simulink model "test"  (R2021a)
settings: Solver=FixedStepAuto  StartTime=0.0  StopTime=10  RelTol=1e-3
InitFcn:
  | load('BusDefinitions.mat')
values from neighbouring files (symbols this model uses):
  M = [2.03476350051e-06 9.69056117119e-08 9.69056117119e-08 -1.05662818468e-08 2.03476350051e-06 -9.69056117119e-08 9.69056117119e-08 1.05662818468e-08 2.03476350051e-06 -9.69056117119e-08 -9.69056117119e-08 -1.05662818468e-08 ... (16 elements, 4x4)]    [RSdata_Kalman.mat]
undefined symbols (not defined in the file or in its folder): codertarget, Ts, W
settings Model: ExtModeTrigDuration=80  Creator=tomwh  LastModifiedBy=tomwh
settings SolverCC: AlgebraicLoopSolver=TrustRegion
settings OptimizationCC: PassReuseOutputArgsThreshold=0  MaxStackSize=64
settings DebuggingCC: ParameterTunabilityLossMsg=error  SFMachineParentedDataDiag=warning  ArithmeticOperatorsInVariantConditions=warning
settings HardwareCC: ProdBitPerPointer=32  ProdBitPerSizeT=32  ProdBitPerPtrDiffT=32  ProdLargestAtomicInteger=Long  ProdWordSize=32  ProdHWDeviceType=ARM Compatible->ARM 9  UseEmbeddedCoderFeatures=off
settings SFSimCC: SimUseLocalCustomCode=off  MATLABDynamicMemAlloc=off
settings RTWCC: SystemTargetFile=ert.tlc  HardwareBoard=PARROT Mambo  TLCOptions="-aInlineSetEventsForThisBaseRateFcn=TLC_FALSE -aSuppressMultiTaskScheduler=TLC_FALSE   -aRateBasedStepFcn=1"  TemplateMakefile=ert_default_tmf  GenerateReport=on  RTWUseLocalCustomCode=off  Toolchain=Sourcery G++ Lite GNU Toolchain for Drones  LaunchReport=on
settings CodeAppCC: ForceParamTrailComments=on  OperatorAnnotations=on  StateflowObjectComments=on
settings ERTTargetCC: ERTCustomFileBanners=off  MatFileLogging=on  SupportContinuousTime=on  SupportNonInlinedSFcns=on  RemoveResetFunc=off  ModelStepFunctionPrototypeControlCompliant=off

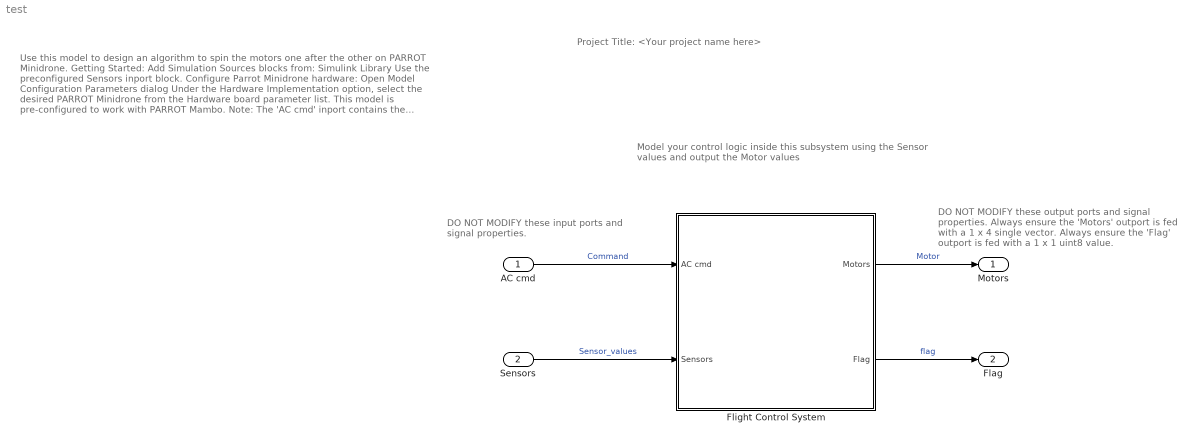
== system test ==
  note: Model your control logic inside this subsystem
      | using the Sensor values and output the
      | Motor values
  note: DO NOT MODIFY these output ports
      | and signal properties.
      |
      |
      |
      | Always ensure the 'Motors' outport
      | is fed with a 1 x 4 single vector.
      |
      |
      |
      |
      |
      | Always ensure the 'Flag' outport is
      | fed with a 1 x 1 uint8 value.
  note: DO NOT MODIFY these input
      | ports and signal properties.
  note: Use this model to design an algorithm to spin the motors one
      | after the other on PARROT Minidrone.
      |
      | Getting Started:
      |
      | Add Simulation Sources blocks from:
      | Simulink Library
      | Use the preconfigured Sensors inport block.
      |
      | Configure Parrot Minidrone hardware:
      |
      | Open Model Configuration Parameters dialog
      |
      | Under the Hardware Implementation option, select the desired
      | PARROT Minidrone from the Hardware board parameter list.
      |
      | This model is pre-configured to work with PARROT Mambo.
      |
      | Note:
      |
      | The 'AC cmd' inport contains the position and orientation
      | reference signals information.
      | The 'Sensors' inport contains data from accelerometer,
      | gyroscope, ultrasonic, pressure and optical flow data.
      | The 'Flag' outport can be used to model an error condition
      | which stops the drone.
      | The 'Motors' outport is fed with the speed values of the 4 motors.
      | Learn more:
      |
      | Simulink Subsystem
      | Simulink Buses
  note: Project Title: <Your project name here>
  AC cmd : Inport  OutDataTypeStr=Bus: CommandBus  BusOutputAsStruct=on
  Sensors : Inport  Port=2  OutDataTypeStr=Bus: SensorsBus  BusOutputAsStruct=on
  Flight Control System : Subsystem  InitFcn=codertarget.parrot.internal.fcsSubsystemCallback(gcb);
  Motors : Outport  OutDataTypeStr=single  PortDimensions=[1 4]  VectorParamsAs1DForOutWhenUnconnected=off
  Flag : Outport  Port=2  OutDataTypeStr=uint8  PortDimensions=1  VectorParamsAs1DForOutWhenUnconnected=off
  wires:
  Flight Control System/1(Motors) -> Motors/1  "Motor"
  AC cmd/1 -> Flight Control System/1(AC cmd)  "Command"
  Sensors/1 -> Flight Control System/2(Sensors)  "Sensor_values"
  Flight Control System/2(Flag) -> Flag/1  "flag"

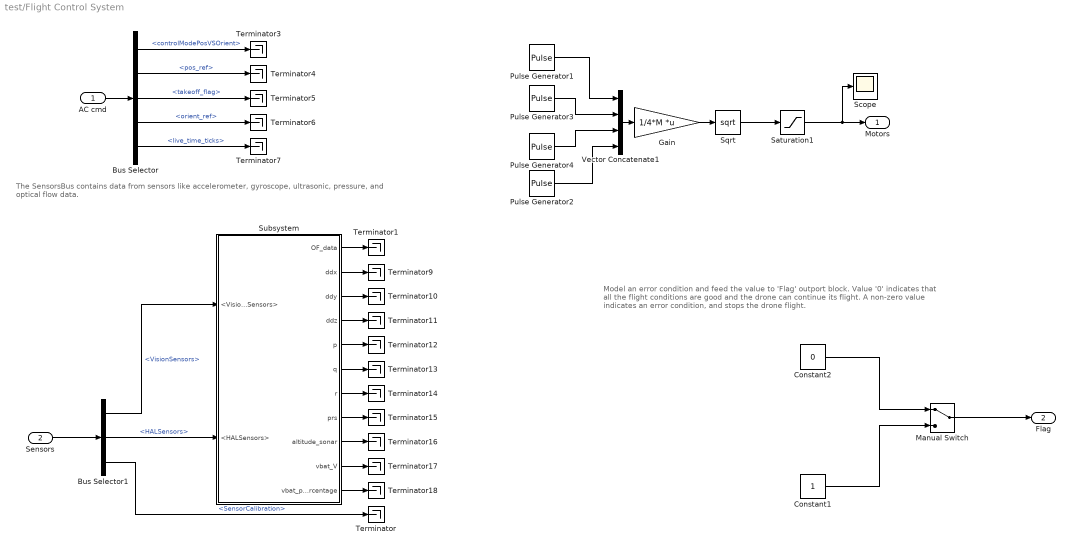
== system test/Flight Control System ==
  note: Model an error condition and feed the value to 'Flag' outport block.
      | Value '0' indicates that all the flight conditions are good and the drone
      | can continue its flight.
      | A non-zero value indicates an error condition, and stops the drone
      | flight.
  note: The SensorsBus contains data from sensors like
      | accelerometer, gyroscope, ultrasonic, pressure,
      | and optical flow data.
  AC cmd : Inport
  Sensors : Inport  Port=2
  Bus Selector : BusSelector  OutputSignals=controlModePosVSOrient,pos_ref,takeoff_flag,orient_ref,live_time_ticks
  Bus Selector1 : BusSelector  OutputSignals=VisionSensors,HALSensors,SensorCalibration
  Constant1 : Constant  OutDataTypeStr=uint8
  Constant2 : Constant  Value=0  OutDataTypeStr=uint8
  Gain : Gain  Gain=1/4*M  Multiplication=Matrix(K*u)
  Manual Switch : ManualSwitch
  Pulse Generator1 : DiscretePulseGenerator  Amplitude=W(1)  Period=1600  PulseWidth=400  SampleTime=Ts
  Pulse Generator2 : DiscretePulseGenerator  Amplitude=W(4)  Period=1600  PulseWidth=400  PhaseDelay=1200  SampleTime=Ts
  Pulse Generator3 : DiscretePulseGenerator  Amplitude=W(2)  Period=1600  PulseWidth=400  PhaseDelay=400  SampleTime=Ts
  Pulse Generator4 : DiscretePulseGenerator  Amplitude=W(3)  Period=1600  PulseWidth=400  PhaseDelay=800  SampleTime=Ts
  Saturation1 : Saturate  UpperLimit=500  LowerLimit=0  OutDataTypeStr=single
  Scope : Scope
  Sqrt : Sqrt  SaturateOnIntegerOverflow=on
  Subsystem : Subsystem
  Terminator{,1,3..7,9..18} (17 alike) : Terminator
  Vector Concatenate1 : Concatenate  NumInputs=4
  Motors : Outport  VectorParamsAs1DForOutWhenUnconnected=off
  Flag : Outport  Port=2  VectorParamsAs1DForOutWhenUnconnected=off
  wires:
  AC cmd/1 -> Bus Selector/1
  Sensors/1 -> Bus Selector1/1
  Bus Selector/1 -> Terminator3/1  "<controlModePosVSOrient>"
  Bus Selector/2 -> Terminator4/1  "<pos_ref>"
  Bus Selector/3 -> Terminator5/1  "<takeoff_flag>"
  Bus Selector/4 -> Terminator6/1  "<orient_ref>"
  Bus Selector/5 -> Terminator7/1  "<live_time_ticks>"
  Manual Switch/1 -> Flag/1
  Constant2/1 -> Manual Switch/1
  Constant1/1 -> Manual Switch/2
  Pulse Generator1/1 -> Vector Concatenate1/1
  Pulse Generator2/1 -> Vector Concatenate1/4
  Pulse Generator3/1 -> Vector Concatenate1/2
  Pulse Generator4/1 -> Vector Concatenate1/3
  Saturation1/1 -> Scope/1, Motors/1
  Bus Selector1/1 -> Subsystem/1(<VisionSensors>)  "<VisionSensors>"
  Bus Selector1/2 -> Subsystem/2(<HALSensors>)  "<HALSensors>"
  Bus Selector1/3 -> Terminator/1  "<SensorCalibration>"
  Subsystem/1(OF_data) -> Terminator1/1
  Subsystem/2(ddx) -> Terminator9/1
  Subsystem/3(ddy) -> Terminator10/1
  Subsystem/4(ddz) -> Terminator11/1
  Subsystem/5(p) -> Terminator12/1
  Subsystem/7(r) -> Terminator14/1
  Subsystem/8(prs) -> Terminator15/1
  Subsystem/9(altitude_sonar) -> Terminator16/1
  Subsystem/10(vbat_V) -> Terminator17/1
  Subsystem/11(vbat_percentage) -> Terminator18/1
  Subsystem/6(q) -> Terminator13/1
  Vector Concatenate1/1 -> Gain/1
  Gain/1 -> Sqrt/1
  Sqrt/1 -> Saturation1/1

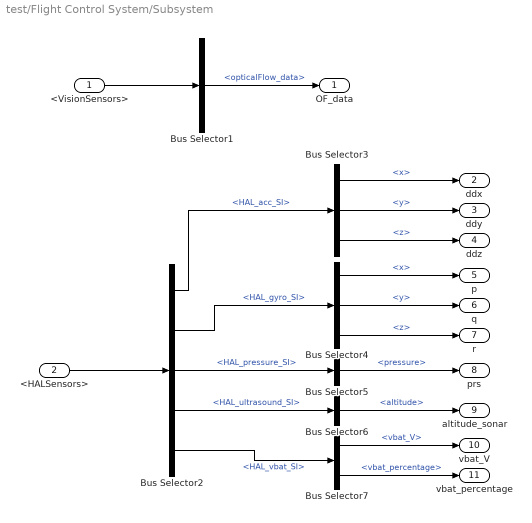
== system test/Flight Control System/Subsystem ==
  <VisionSensors> : Inport
  <HALSensors> : Inport  Port=2
  Bus Selector1 : BusSelector  OutputSignals=opticalFlow_data
  Bus Selector2 : BusSelector  OutputSignals=HAL_acc_SI,HAL_gyro_SI,HAL_pressure_SI,HAL_ultrasound_SI,HAL_vbat_SI
  Bus Selector3 : BusSelector  OutputSignals=x,y,z
  Bus Selector4 : BusSelector  OutputSignals=x,y,z
  Bus Selector5 : BusSelector  OutputSignals=pressure
  Bus Selector6 : BusSelector  OutputSignals=altitude
  Bus Selector7 : BusSelector  OutputSignals=vbat_V,vbat_percentage
  OF_data : Outport  VectorParamsAs1DForOutWhenUnconnected=off
  ddx : Outport  Port=2  VectorParamsAs1DForOutWhenUnconnected=off
  ddy : Outport  Port=3  VectorParamsAs1DForOutWhenUnconnected=off
  ddz : Outport  Port=4  VectorParamsAs1DForOutWhenUnconnected=off
  p : Outport  Port=5  VectorParamsAs1DForOutWhenUnconnected=off
  q : Outport  Port=6  VectorParamsAs1DForOutWhenUnconnected=off
  r : Outport  Port=7  VectorParamsAs1DForOutWhenUnconnected=off
  prs : Outport  Port=8  VectorParamsAs1DForOutWhenUnconnected=off
  altitude_sonar : Outport  Port=9  VectorParamsAs1DForOutWhenUnconnected=off
  vbat_V : Outport  Port=10  VectorParamsAs1DForOutWhenUnconnected=off
  vbat_percentage : Outport  Port=11  VectorParamsAs1DForOutWhenUnconnected=off
  wires:
  <VisionSensors>/1 -> Bus Selector1/1
  <HALSensors>/1 -> Bus Selector2/1
  Bus Selector1/1 -> OF_data/1  "<opticalFlow_data>"
  Bus Selector2/1 -> Bus Selector3/1  "<HAL_acc_SI>"
  Bus Selector2/2 -> Bus Selector4/1  "<HAL_gyro_SI>"
  Bus Selector2/3 -> Bus Selector5/1  "<HAL_pressure_SI>"
  Bus Selector2/4 -> Bus Selector6/1  "<HAL_ultrasound_SI>"
  Bus Selector2/5 -> Bus Selector7/1  "<HAL_vbat_SI>"
  Bus Selector3/1 -> ddx/1  "<x>"
  Bus Selector3/2 -> ddy/1  "<y>"
  Bus Selector3/3 -> ddz/1  "<z>"
  Bus Selector4/2 -> q/1  "<y>"
  Bus Selector4/1 -> p/1  "<x>"
  Bus Selector4/3 -> r/1  "<z>"
  Bus Selector5/1 -> prs/1  "<pressure>"
  Bus Selector6/1 -> altitude_sonar/1  "<altitude>"
  Bus Selector7/1 -> vbat_V/1  "<vbat_V>"
  Bus Selector7/2 -> vbat_percentage/1  "<vbat_percentage>"
